simulink model "VVIR"  (R2021b)
settings: Solver=FixedStepAuto  StartTime=0.0  StopTime=inf  FixedStep=0.001  RelTol=1e-3  EnableMultiTasking=on
undefined symbols (not defined in the file): D1, D10, D11, D12, D13, D2, D3, D4, D5, D7, D8, D9, PTA0, PTA1, PTA2, PTB23, PTB9, PTC17, PTC3, PTC4, PTD0, PTD1, PTD2, PTD3
libraries: frdmk64flib x13, simulink x5
settings Model: ExtModeTrigDuration=5  Creator=12268  LastModifiedBy=Aaron
settings SolverCC: AlgebraicLoopSolver=TrustRegion
settings OptimizationCC: EnhancedBackFolding=on  PassReuseOutputArgsAs=Individual arguments  ZeroExternalMemoryAtStartup=off  ZeroInternalMemoryAtStartup=off  MaxStackSize=64  OptimizeBlockOrder=speed  DifferentSizesBufferReuse=on  OptimizationCustomize=off  EfficientTunableParamExpr=on
settings DebuggingCC: ParameterTunabilityLossMsg=error  SFMachineParentedDataDiag=warning
settings HardwareCC: ProdBitPerPointer=32  ProdBitPerSizeT=32  ProdBitPerPtrDiffT=32  ProdLargestAtomicInteger=Long  ProdLargestAtomicFloat=Double  ProdWordSize=32  ProdHWDeviceType=ARM Compatible->ARM Cortex
settings SFSimCC: MATLABDynamicMemAlloc=off
settings RTWCC: Description=Embedded Coder  SystemTargetFile=ert.tlc  HardwareBoard=NXP FRDM-K64F  TLCOptions="-aInlineSetEventsForThisBaseRateFcn=TLC_FALSE -aSuppressMultiTaskScheduler=TLC_FALSE  -aRateBasedStepFcn=0"  TemplateMakefile=ert_default_tmf  Toolchain=GNU Tools for ARM Embedded Processors
settings CodeAppCC: ForceParamTrailComments=on  IgnoreCustomStorageClasses=off  OperatorAnnotations=on  SimulinkDataObjDesc=on  SFDataObjDesc=on  InsertBlockDesc=on

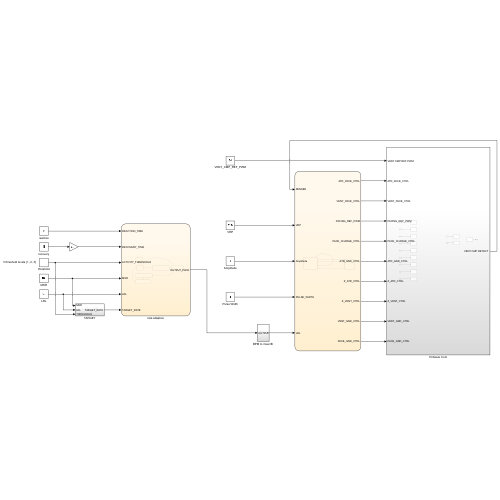
[thumbnail: Simulink's stored preview of the top-level diagram]
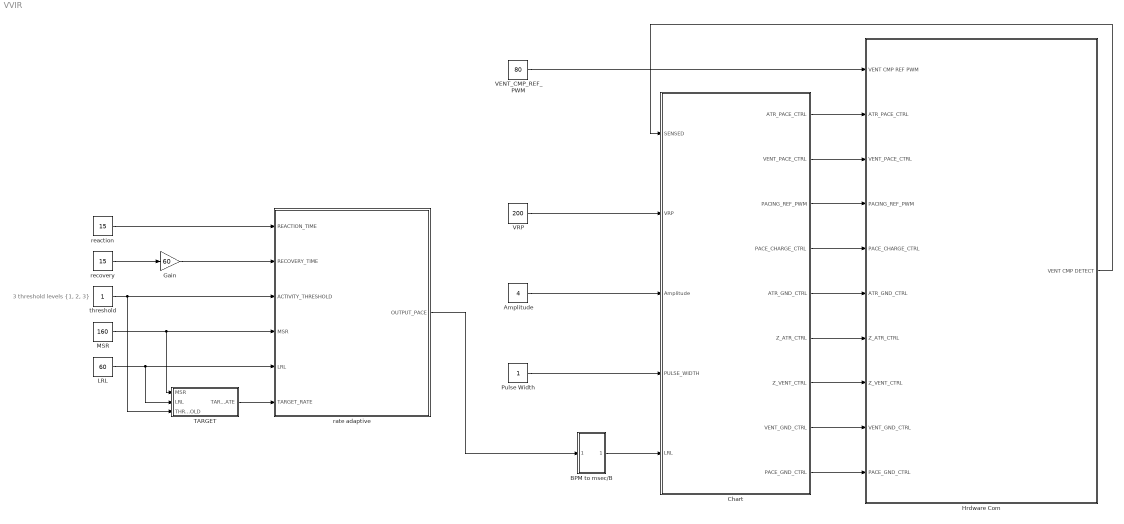
== system VVIR ==
  note: 3 threshold levels {1, 2, 3}
  Amplitude : Constant  Value=4  OutDataTypeStr=double
  "BPM to msec/B " : Subsystem
  Chart : Stateflow chart  TreatAsAtomicUnit=on
  Gain : Gain  Gain=60
  Hrdware Com : Subsystem
  LRL : Constant  Value=60
  MSR : Constant  Value=160
  Pulse Width : Constant  OutDataTypeStr=uint16
  TARGET : Subsystem
  VENT_CMP_REF_PWM : Constant  Value=80  OutDataTypeStr=double
  VRP : Constant  Value=200  OutDataTypeStr=uint16
  rate adaptive : Stateflow chart  TreatAsAtomicUnit=on
      settings: PortSchema="{\"entries\":[{\"content\":{\"sides\":[{\"content\":{\"connectorIds\":[\"In3\",\"In4\",\"In5\",\"In1\",\"In2\",\"In6\"]},\"type\":\"ConnectorPlacement.EquallySpacedRectSide\",\"uuid\":\"d3aa46b7-da68-4733-bd03-102d604fce17\"},{\"content\":{\"connectorIds\":[\"Out1\"],\"side\":\"RIGHT\"},\"type\":\"ConnectorPlacement.EquallySpacedRectSide\",\"uuid\":\"afbb636e-6b76-41fa-bb75-ca0d3f63044e\"},{\"content\":{\"connectorIds\":[],\"side\":\"TOP\"},\"type\":\"ConnectorPlacement.EquallySpacedRectSide\",\"uuid\":\"40571637-2e0f-45fd-89f0-6c332ecbd683\"}]},\"type\":\"ConnectorPlacement.EquallySpacedConnector\",\"uuid\":\"5e4e3dcb-fc0d-40cc-8fd4-4ca115cadd01\"}],\"packageUris\":[\"http://schema.mathworks.com/mf0/Connector/R2020b\"],\"version\":\"1.0\"}"
  reaction : Constant  Value=15  OutDataTypeStr=double
  recovery : Constant  Value=15  OutDataTypeStr=double
  threshold : Constant  OutDataTypeStr=single
  wires:
  Amplitude/1 -> Chart/3(Amplitude)
  Pulse Width/1 -> Chart/4(PULSE_WIDTH)
  "BPM to msec/B "/1(Out1) -> Chart/5(LRL)
  Chart/1(ATR_PACE_CTRL) -> Hrdware Com/2(ATR_PACE_CTRL)
  Chart/2(VENT_PACE_CTRL) -> Hrdware Com/3(VENT_PACE_CTRL)
  Chart/3(PACING_REF_PWM) -> Hrdware Com/4(PACING_REF_PWM)
  Chart/4(PACE_CHARGE_CTRL) -> Hrdware Com/5(PACE_CHARGE_CTRL)
  Chart/5(ATR_GND_CTRL) -> Hrdware Com/6(ATR_GND_CTRL)
  Chart/6(Z_ATR_CTRL) -> Hrdware Com/7("Z_ATR_CTRL ")
  Chart/7(Z_VENT_CTRL) -> Hrdware Com/8("Z_VENT_CTRL ")
  Chart/8(VENT_GND_CTRL) -> Hrdware Com/9(VENT_GND_CTRL)
  Chart/9(PACE_GND_CTRL) -> Hrdware Com/10(PACE_GND_CTRL)
  Hrdware Com/1("VENT CMP DETECT ") -> Chart/1(SENSED)
  VENT_CMP_REF_PWM/1 -> Hrdware Com/1(VENT CMP REF PWM)
  VRP/1 -> Chart/2(VRP)
  threshold/1 -> TARGET/3(THRESHOLD), rate adaptive/5(ACTIVITY_THRESHOLD)
  TARGET/1(TARGET_RATE) -> rate adaptive/6(TARGET_RATE)
  MSR/1 -> TARGET/1(MSR), rate adaptive/1(MSR)
  reaction/1 -> rate adaptive/3(REACTION_TIME)
  Gain/1 -> rate adaptive/4(RECOVERY_TIME)
  LRL/1 -> rate adaptive/2(LRL), TARGET/2(LRL)
  recovery/1 -> Gain/1
  rate adaptive/1(OUTPUT_PACE) -> "BPM to msec/B "/1(OUTPUT_PACE)

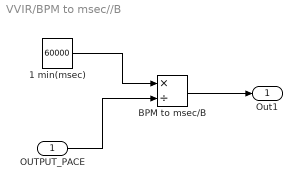
== system VVIR/BPM to msec//B  ==
  OUTPUT_PACE : Inport
  1 min(msec) : Constant  Value=60000  OutDataTypeStr=double
  "BPM to msec/B " : Product  Inputs=*/  OutDataTypeStr=uint16  RndMeth=Nearest
  Out1 : Outport
  wires:
  1 min(msec)/1 -> "BPM to msec/B "/1
  "BPM to msec/B "/1 -> Out1/1
  OUTPUT_PACE/1 -> "BPM to msec/B "/2

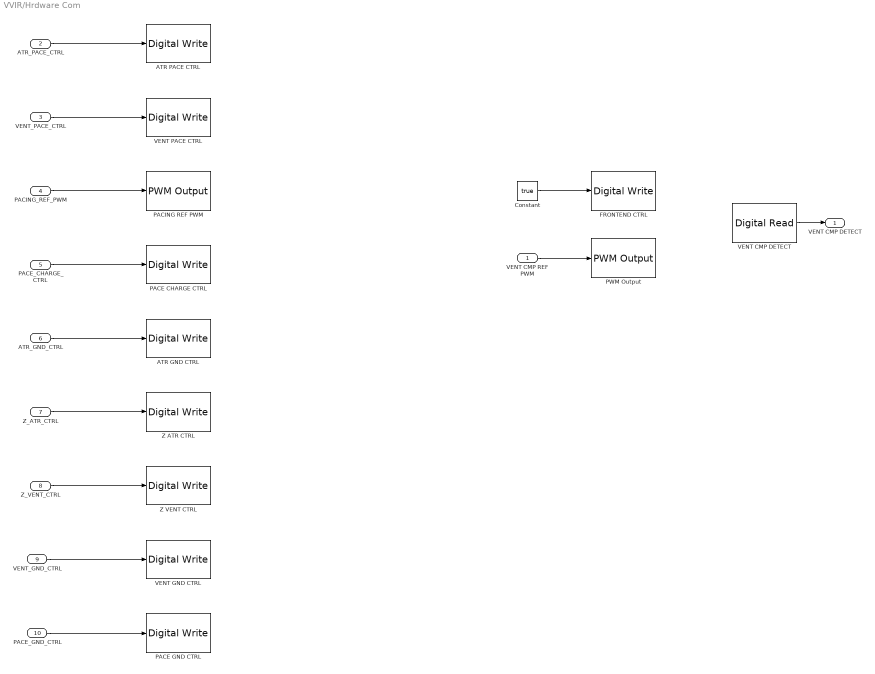
== system VVIR/Hrdware Com ==
  VENT CMP REF PWM : Inport
  ATR_PACE_CTRL : Inport  Port=2
  VENT_PACE_CTRL : Inport  Port=3
  PACING_REF_PWM : Inport  Port=4
  PACE_CHARGE_CTRL : Inport  Port=5
  ATR_GND_CTRL : Inport  Port=6
  "Z_ATR_CTRL " : Inport  Port=7
  "Z_VENT_CTRL " : Inport  Port=8
  VENT_GND_CTRL : Inport  Port=9
  PACE_GND_CTRL : Inport  Port=10
  "ATR GND CTRL " : frdmk64flib/Digital Write  Whichpin=PTD2 (D11)
  ATR PACE CTRL : frdmk64flib/Digital Write  Whichpin=PTA0 (D8)
  Constant : Constant  Value=true  OutDataTypeStr=boolean
  FRONTEND CTRL : frdmk64flib/Digital Write  Whichpin=PTD1 (D13)
  PACE CHARGE CTRL : frdmk64flib/Digital Write  Whichpin=PTB9 (D2)
  PACE GND CTRL : frdmk64flib/Digital Write  Whichpin=PTD0 (D10)
  PACING REF PWM : frdmk64flib/PWM Output  Whichpin=PTA2 (D5)  InitialFrequency=2000  InitialDutyCycle=0
  PWM Output : frdmk64flib/PWM Output  Whichpin=PTA1 (D3)  InitialFrequency=2000  InitialDutyCycle=0
  VENT CMP DETECT : frdmk64flib/Digital Read  Whichpin=PTC17 (D1)  SampleTime=-1
  VENT GND CTRL : frdmk64flib/Digital Write  Whichpin=PTD3 (D12)
  VENT PACE CTRL : frdmk64flib/Digital Write  Whichpin=PTC4 (D9)
  "Z ATR CTRL " : frdmk64flib/Digital Write  Whichpin=PTB23 (D4)
  "Z VENT CTRL " : frdmk64flib/Digital Write  Whichpin=PTC3 (D7)
  "VENT CMP DETECT " : Outport  OutDataTypeStr=boolean  PortDimensions=1
  wires:
  ATR_PACE_CTRL/1 -> ATR PACE CTRL/1
  VENT_PACE_CTRL/1 -> VENT PACE CTRL/1
  PACING_REF_PWM/1 -> PACING REF PWM/1
  PACE_CHARGE_CTRL/1 -> PACE CHARGE CTRL/1
  ATR_GND_CTRL/1 -> "ATR GND CTRL "/1
  "Z_ATR_CTRL "/1 -> "Z ATR CTRL "/1
  "Z_VENT_CTRL "/1 -> "Z VENT CTRL "/1
  VENT_GND_CTRL/1 -> VENT GND CTRL/1
  PACE_GND_CTRL/1 -> PACE GND CTRL/1
  Constant/1 -> FRONTEND CTRL/1
  VENT CMP DETECT/1 -> "VENT CMP DETECT "/1
  VENT CMP REF PWM/1 -> PWM Output/1

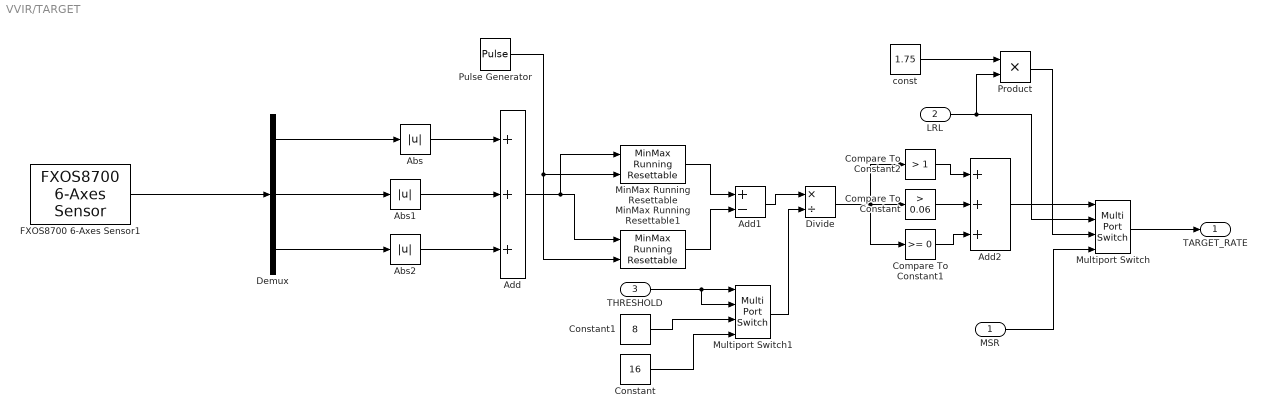
== system VVIR/TARGET ==
  MSR : Inport
  LRL : Inport  Port=2
  THRESHOLD : Inport  Port=3
  Abs : Abs
  Abs1 : Abs
  Abs2 : Abs
  Add : Sum  Inputs=+++
  Add1 : Sum  Inputs=+-
  Add2 : Sum  Inputs=+++
  Compare To Constant : simulink/Logic and Bit Operations/Compare To Constant  relop=>  const=0.06  OutDataTypeStr=uint8
  Compare To Constant1 : simulink/Logic and Bit Operations/Compare To Constant  relop=>=  const=0  OutDataTypeStr=uint8
  Compare To Constant2 : simulink/Logic and Bit Operations/Compare To Constant  relop=>  const=1  OutDataTypeStr=uint8
  Constant : Constant  Value=16  OutDataTypeStr=single
  Constant1 : Constant  Value=8  OutDataTypeStr=single
  Demux : Demux  Outputs=3
  Divide : Product  Inputs=*/
  FXOS8700 6-Axes Sensor1 : frdmk64flib/FXOS8700 6-Axes Sensor  Activesensor=Accelerometer only  ODR=800Hz  HybridODR=400Hz  Accelfullrange=-2g to +2g  SampleTime=-1
  MinMax Running Resettable : simulink/Math Operations/MinMax Running Resettable  Function=max  vinit=1
  MinMax Running Resettable1 : simulink/Math Operations/MinMax Running Resettable  Function=min  vinit=1
  Multiport Switch : MultiPortSwitch  OutDataTypeStr=double
  Multiport Switch1 : MultiPortSwitch
  Product : Product
  Pulse Generator : DiscretePulseGenerator  PulseType=Time based  PulseWidth=2.5
  const : Constant  Value=1.75
  TARGET_RATE : Outport
  wires:
  Compare To Constant/1 -> Add2/2
  Multiport Switch/1 -> TARGET_RATE/1
  Compare To Constant1/1 -> Add2/3
  Add2/1 -> Multiport Switch/1
  LRL/1 -> Product/2, Multiport Switch/2
  Product/1 -> Multiport Switch/3
  Abs2/1 -> Add/3
  Add/1 -> MinMax Running Resettable1/1, MinMax Running Resettable/1
  MinMax Running Resettable1/1 -> Add1/2
  Demux/2 -> Abs1/1
  Demux/3 -> Abs2/1
  Compare To Constant2/1 -> Add2/1
  MinMax Running Resettable/1 -> Add1/1
  Demux/1 -> Abs/1
  Pulse Generator/1 -> MinMax Running Resettable1/2, MinMax Running Resettable/2
  Abs/1 -> Add/1
  Abs1/1 -> Add/2
  FXOS8700 6-Axes Sensor1/1 -> Demux/1
  MSR/1 -> Multiport Switch/4
  const/1 -> Product/1
  Divide/1 -> Compare To Constant/1, Compare To Constant2/1, Compare To Constant1/1
  Add1/1 -> Divide/1
  Multiport Switch1/1 -> Divide/2
  THRESHOLD/1 -> Multiport Switch1/2, Multiport Switch1/1
  Constant/1 -> Multiport Switch1/4
  Constant1/1 -> Multiport Switch1/3

== stateflow chart VVIR/Chart ==
  state Charging_and_Discharging
    entry:
    PACE_GND_CTRL=true;
    ATR_PACE_CTRL=false;
    VENT_PACE_CTRL=false;
    PACING_REF_PWM=uint8(Amplitude*20);
    PACE_CHARGE_CTRL=true;
    Z_ATR_CTRL=false;
    Z_VENT_CTRL=false;
    ATR_GND_CTRL=false;
    VENT_GND_CTRL=true;
  state V_Pacing
    entry:
    PACE_CHARGE_CTRL=false;
    PACE_GND_CTRL=true;
    ATR_GND_CTRL=false;
    Z_ATR_CTRL=false;
    Z_VENT_CTRL=false;
    VENT_GND_CTRL=false;
    ATR_PACE_CTRL=false;
    VENT_PACE_CTRL=true;
    PACED=true;
  (junction 69) -> Charging_and_Discharging [order 1] : [SENSED==true]{PACED=false}
  (default) -> Charging_and_Discharging
  Charging_and_Discharging -> (junction 69) [order 2] : after(VRP, msec)[PACED==false]
  (junction 69) -> V_Pacing [order 2] : after(LRL-VRP, msec)
  (junction 70) -> V_Pacing [order 2] : after(LRL-VRP, msec)
  Charging_and_Discharging -> (junction 70) [order 1] : after(VRP-PULSE_WIDTH, msec)[PACED==true]
  (junction 70) -> Charging_and_Discharging [order 1] : [SENSED==true]{PACED=false}
  V_Pacing -> Charging_and_Discharging : after(PULSE_WIDTH, msec)
  data: SENSED input boolean; VRP input uint16; ATR_PACE_CTRL output boolean; VENT_PACE_CTRL output boolean; PACING_REF_PWM output uint8; Amplitude input double; PACE_CHARGE_CTRL output boolean; ATR_GND_CTRL output boolean; Z_ATR_CTRL output boolean; Z_VENT_CTRL output boolean; VENT_GND_CTRL output boolean; PACE_GND_CTRL output boolean; PULSE_WIDTH input uint16; LRL input uint16; PACED local boolean =false

== stateflow chart VVIR/rate adaptive ==
  state start
    entry:
    OUTPUT_PACE = LRL;
  state IDLE
  state increase_pace
    entry:
    OUTPUT_PACE = OUTPUT_PACE + increment;
  state calculate_increment
    entry:
    increment = 2.5*(TARGET_RATE-OUTPUT_PACE) / REACTION_TIME;
  state calculate_decrement
    entry:
    decrement = (OUTPUT_PACE - TARGET_RATE) / RECOVERY_TIME;
  state decrease_pace
    entry:
    OUTPUT_PACE = OUTPUT_PACE - decrement;
  (default) -> start
  increase_pace -> IDLE [order 1] : [OUTPUT_PACE == TARGET_RATE]
  start -> IDLE
  calculate_increment -> increase_pace
  decrease_pace -> IDLE : after(500,msec)
  IDLE -> calculate_increment [order 1] : [TARGET_RATE > OUTPUT_PACE]
  IDLE -> calculate_decrement [order 2] : [TARGET_RATE < OUTPUT_PACE]
  increase_pace -> calculate_decrement [order 3] : [TARGET_RATE < OUTPUT_PACE]
  increase_pace -> increase_pace [order 2] : after(1,sec)
  calculate_decrement -> decrease_pace
  data: MSR input double; LRL input double; REACTION_TIME input double; RECOVERY_TIME input double; ACTIVITY_THRESHOLD input single; OUTPUT_PACE output double; TARGET_RATE input double; decrement local double; increment local double
